simulink model "test03"  (R2021a)
settings: Solver=VariableStepAuto  StartTime=0.0  StopTime=10  RelTol=1e-3
libraries: HORTISIM x3
settings Model: Creator=djoroya  LastModifiedBy=djoroya
settings DebuggingCC: UnconnectedInputMsg=none  UnconnectedOutputMsg=none  UnconnectedLineMsg=none

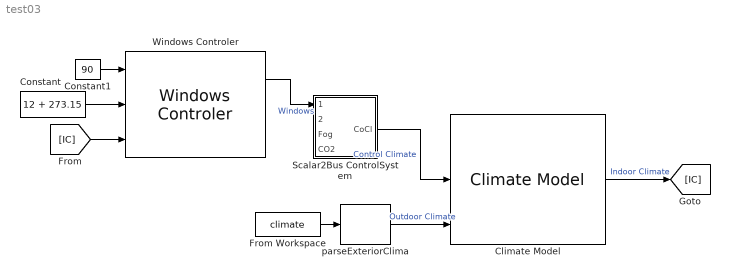
== system test03 ==
  Climate Model : HORTISIM/Climate/Models/Climate Model  params=params  x0=cic
      settings: SourceProductName=Horti Simulator
  Constant : Constant  Value=12 + 273.15
  Constant1 : Constant  Value=90
  From Workspace : FromWorkspace  VariableName=climate
  Scalar2Bus ControlSystem : Subsystem  AncestorBlock=|
      | HORTISIM/Other 
      | Functions/Scalar2Bus 
      | ControlSystem
  Windows Controler : HORTISIM/Climate/Controls/Windows Controler  MaxT100=5
      settings: SourceProductName=Horti Simulator
  parseExteriorClima : HORTISIM/Other  Functions/parseExteriorClima  SystemSampleTime=-1  VariantActivationTime=update diagram  Latency=0  AutoFrameSizeCalculation=off
      settings: SourceProductName=Horti Simulator
  wires:
  From Workspace/1 -> parseExteriorClima/1
  parseExteriorClima/1 -> Climate Model/3  "Outdoor Climate"
  Climate Model/1 -> [IC]  "Indoor Climate"
  Scalar2Bus ControlSystem/1(CoCl) -> Climate Model/2  "Control Climate"
  [IC] -> Windows Controler/3
  Windows Controler/1 -> Scalar2Bus ControlSystem/1(Windows)  "Windows"
  Constant/1 -> Windows Controler/2
  Constant1/1 -> Windows Controler/1

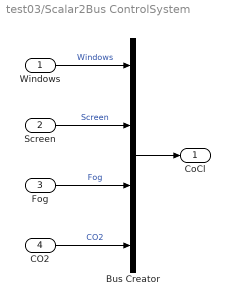
== system test03/Scalar2Bus ControlSystem ==
  Windows : Inport
  Screen : Inport  Port=2
  Fog : Inport  Port=3
  CO2 : Inport  Port=4
  Bus Creator : BusCreator  Inputs=4
  CoCl : Outport
  wires:
  Fog/1 -> Bus Creator/3  "Fog"
  CO2/1 -> Bus Creator/4  "CO2"
  Windows/1 -> Bus Creator/1  "Windows"
  Bus Creator/1 -> CoCl/1
  Screen/1 -> Bus Creator/2  "Screen"
